simulink model "c8mnlf1"  (R2022a)
settings: Solver=ode15s  StartTime=0.0  StopTime=4  RelTol=1e-8  EnableMultiTasking=on
PreLoadFcn:
  | ww=[1e-4 1e4]; N=11;
libraries: cstblocks x4
settings Model: Creator=yj  LastModifiedBy=xuedi
settings SolverCC: AlgebraicLoopSolver=TrustRegion
settings DataIOCC: SaveFormat=Array  SignalLoggingSaveFormat=ModelDataLogs  ReturnWorkspaceOutputs=off  SignalLoggingName=sigsOut
settings OptimizationCC: ExpressionDepthLimit=2147483647  InitFltsAndDblsToZero=on  LifeSpan=inf
settings DebuggingCC: AlgebraicLoopMsg=none  SaveWithParameterizedLinksMsg=none  UnderspecifiedInitializationDetection=Classic  MergeDetectMultiDrivingBlocksExec=none  SignalResolutionControl=TryResolveAllWithWarning  MultiTaskDSMMsg=warning  MultiTaskCondExecSysMsg=none  FcnCallInpInsideContextMsg=warning  UnconnectedInputMsg=warning  UnconnectedOutputMsg=warning  UnconnectedLineMsg=warning  StateNameClashWarn=warning  SFUnexpectedBacktrackingDiag=warning  SFNoUnconditionalDefaultTransitionDiag=warning  SFExecutionAtInitializationDiag=none  SFMachineParentedDataDiag=warning  ArithmeticOperatorsInVariantConditions=warning
settings HardwareCC: ProdBitPerPointer=32  ProdBitPerSizeT=32  ProdBitPerPtrDiffT=32  ProdLargestAtomicFloat=None  ProdIntDivRoundTo=Undefined  ProdEndianess=Unspecified  ProdWordSize=32  ProdHWDeviceType=32-bit Generic  TargetUnknown=on
settings ModelReferenceCC: PropagateSignalLabelsOutOfModel=off
settings SFSimCC: SimUseLocalCustomCode=off  CustomCodeUndefinedFunction=UseInterfaceOnly
settings RTWCC: RTWUseLocalCustomCode=off  DLArmComputeVersion=19.05
settings CodeAppCC: StateflowObjectComments=on
settings GRTTargetCC: TargetLangStandard=C89/C90 (ANSI)  CombineOutputUpdateFcns=off  GRTInterface=on
settings ConfigComp: CovMetricSettings=dw  CovSaveCumulativeToWorkspaceVar=on  CovSaveSingleToWorkspaceVar=on  CovExternalEMLEnable=off

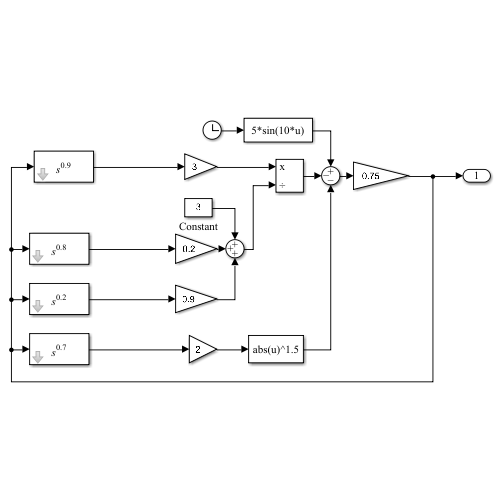
[thumbnail: Simulink's stored preview of the top-level diagram]
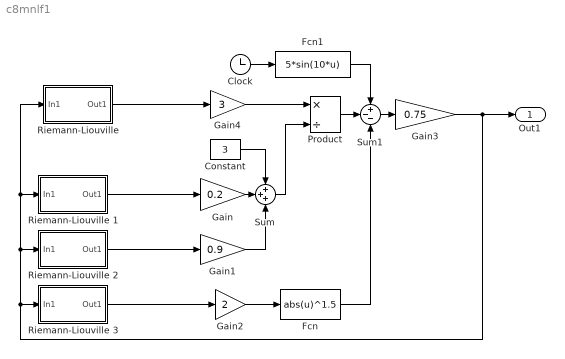
== system c8mnlf1 ==
  Clock : Clock
  Constant : Constant  Value=3
  Fcn : Fcn  Expr=abs(u)^1.5
  Fcn1 : Fcn  Expr=5*sin(10*u)
  Gain : Gain  Gain=0.2  SaturateOnIntegerOverflow=on  OutDataTypeStr=Inherit: Same as input  ParamDataTypeStr=Inherit: Same as input
  Gain1 : Gain  Gain=0.9  SaturateOnIntegerOverflow=on  OutDataTypeStr=Inherit: Same as input  ParamDataTypeStr=Inherit: Same as input
  Gain2 : Gain  Gain=2  SaturateOnIntegerOverflow=on  OutDataTypeStr=Inherit: Same as input  ParamDataTypeStr=Inherit: Same as input
  Gain3 : Gain  Gain=0.75  SaturateOnIntegerOverflow=on  OutDataTypeStr=Inherit: Same as input  ParamDataTypeStr=Inherit: Same as input
  Gain4 : Gain  Gain=3  SaturateOnIntegerOverflow=on  OutDataTypeStr=Inherit: Same as input  ParamDataTypeStr=Inherit: Same as input
  Product : Product  Inputs=*/  SaturateOnIntegerOverflow=on  OutDataTypeStr=Inherit: Same as first input
  "Riemann-Liouville " : Subsystem  mask{gam=0.9, ww=ww, n=N, kF1=on, kF=Oustaloup filter}
      mask prompts: gam "Derivative order gamma"; ww "Frequency range [wb,wh]"; n "Apprixmation order"; kF1 "Is a low-pass filter required?"; kF "Filter type"
      mask init:
      | wb=ww(1); wh=ww(2); 
      | if isnumeric(gam), str=['{\its}^{' num2str(gam) '}']; 
      | else, str='{\its}^{\gamma}'; end
      | if kF==1, G=ousta_fod(gam,n,wb,wh);
      | elseif kF==2, G=new_fod(gam,n,wb,wh); 
      | else, G=matsuda_fod(gam,n,wb,wh); end
      | T=1/wh; if kF1==1, G=G*tf(1,[T 1]); end
      mask TypeOptions kF: Oustaloup filter | Modified Oustaloup filter | Matsuda-Fujii filter
      mask Display: disp(str,'texmode','on')
  Riemann-Liouville 1 : Subsystem  mask{gam=0.8, ww=ww, n=N, kF1=on, kF=Oustaloup filter}
      mask prompts: gam "Derivative order gamma"; ww "Frequency range [wb,wh]"; n "Apprixmation order"; kF1 "Is a low-pass filter required?"; kF "Filter type"
      mask init: same as c8mnlf1/Riemann-Liouville 
      mask TypeOptions kF: Oustaloup filter | Modified Oustaloup filter | Matsuda-Fujii filter
      mask Display: disp(str,'texmode','on')
  Riemann-Liouville 2 : Subsystem  mask{gam=0.2, ww=ww, n=N, kF1=on, kF=Oustaloup filter}
      mask prompts: gam "Derivative order gamma"; ww "Frequency range [wb,wh]"; n "Apprixmation order"; kF1 "Is a low-pass filter required?"; kF "Filter type"
      mask init: same as c8mnlf1/Riemann-Liouville 
      mask TypeOptions kF: Oustaloup filter | Modified Oustaloup filter | Matsuda-Fujii filter
      mask Display: disp(str,'texmode','on')
  Riemann-Liouville 3 : Subsystem  mask{gam=0.7, ww=ww, n=N, kF1=on, kF=Oustaloup filter}
      mask prompts: gam "Derivative order gamma"; ww "Frequency range [wb,wh]"; n "Apprixmation order"; kF1 "Is a low-pass filter required?"; kF "Filter type"
      mask init: same as c8mnlf1/Riemann-Liouville 
      mask TypeOptions kF: Oustaloup filter | Modified Oustaloup filter | Matsuda-Fujii filter
      mask Display: disp(str,'texmode','on')
  Sum : Sum  Inputs=+++  SaturateOnIntegerOverflow=on
  Sum1 : Sum  Inputs=+--  SaturateOnIntegerOverflow=on
  Out1 : Outport
  wires:
  Sum/1 -> Product/2
  Gain3/1 -> Riemann-Liouville 2/1(In1), Riemann-Liouville 1/1(In1), "Riemann-Liouville "/1(In1), Riemann-Liouville 3/1(In1), Out1/1
  Fcn1/1 -> Sum1/1
  Product/1 -> Sum1/2
  Sum1/1 -> Gain3/1
  Gain/1 -> Sum/2
  Gain1/1 -> Sum/3
  Constant/1 -> Sum/1
  Gain4/1 -> Product/1
  Gain2/1 -> Fcn/1
  Fcn/1 -> Sum1/3
  "Riemann-Liouville "/1(Out1) -> Gain4/1
  Riemann-Liouville 1/1(Out1) -> Gain/1
  Riemann-Liouville 2/1(Out1) -> Gain1/1
  Riemann-Liouville 3/1(Out1) -> Gain2/1
  Clock/1 -> Fcn1/1

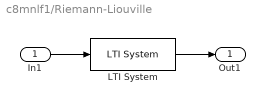
== system c8mnlf1/Riemann-Liouville  ==
  In1 : Inport
  LTI System : cstblocks/LTI System  sys=G  IC=[]
  Out1 : Outport
  wires:
  LTI System/1 -> Out1/1
  In1/1 -> LTI System/1

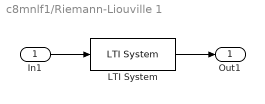
== system c8mnlf1/Riemann-Liouville 1 ==
  In1 : Inport
  LTI System : cstblocks/LTI System  sys=G  IC=[]
  Out1 : Outport
  wires:
  In1/1 -> LTI System/1
  LTI System/1 -> Out1/1

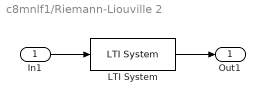
== system c8mnlf1/Riemann-Liouville 2 ==
  In1 : Inport
  LTI System : cstblocks/LTI System  sys=G  IC=[]
  Out1 : Outport
  wires:
  LTI System/1 -> Out1/1
  In1/1 -> LTI System/1

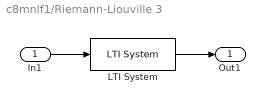
== system c8mnlf1/Riemann-Liouville 3 ==
  In1 : Inport
  LTI System : cstblocks/LTI System  sys=G  IC=[]
  Out1 : Outport
  wires:
  In1/1 -> LTI System/1
  LTI System/1 -> Out1/1
